simulink model "powerwindow04"  (Simulink 10.0)
settings: Solver=ode23tb  StartTime=0.0  StopTime=inf  FixedStep=1e-4  RelTol=1e-2  EnableMultiTasking=on
libraries: powerlib x11, simulink x6, powerwindowlibphys x1, dspquant2 x1
Description:
  | Simulink(R) Power Window Controller With Data Acquisition Effects
  | 
  | In moving to an implementation, additional effects that may affect the control have to be
  | accounted for. This model includes phenomena such as signal conditioning to measure
  | the armature current and quantization of the measurement.
  | 
  | You must install SimMechanics(TM), SimPowerSystems(TM), DSP System Toolbox(TM), and Simulink(R) Fixed Point(TM) to run this power window demo.
settings Model: Creator=The MathWorks Inc.  LastModifiedBy=bhisma  ExtModeAutoUpdateStatusClock=off
settings DataIOCC: LimitDataPoints=on  SignalLoggingSaveFormat=ModelDataLogs  SignalLoggingName=sigsOut
settings OptimizationCC: BooleanDataType=off  ExpressionDepthLimit=2147483647  InitFltsAndDblsToZero=on
settings DebuggingCC: SaveWithParameterizedLinksMsg=none  CheckExecutionContextPreStartOutputMsg=on  CheckExecutionContextRuntimeOutputMsg=on  SignalResolutionControl=TryResolveAllWithWarning  MultiTaskDSMMsg=warning  MultiTaskCondExecSysMsg=none  ParameterPrecisionLossMsg=none  FcnCallInpInsideContextMsg=warning  StateNameClashWarn=warning
settings SFSimCC: SimParseCustomCode=off
settings GRTTargetCC: TargetFcnLib=ansi_tfl_tmw.mat  GeneratePreprocessorConditionals=Disable all
settings ConfigComp: CovExternalEMLEnable=off
settings SimscapeCC: SimscapeNormalizeSystem=off
settings SimMechanicsCC: WarnOnRedundantConstraints=off  VisOnUpdateDiagram=on

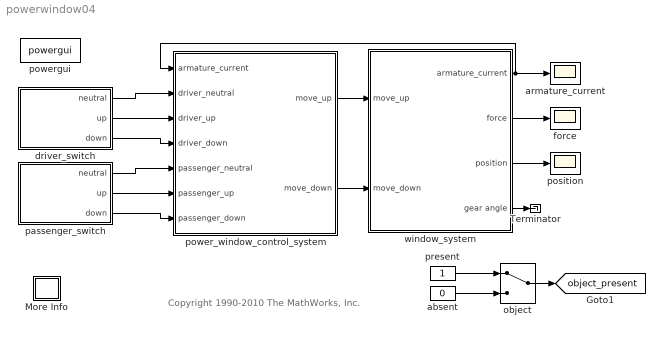
== system powerwindow04 ==
  note: Copyright 1990-2010 The MathWorks, Inc.
  More Info : Subsystem
      settings: OpenFcn=showdemo(bdroot(gcb))
      mask Display: disp('?')
  Terminator : Terminator
  absent : Constant  Value=0
  armature_current : Scope
  driver_switch : Subsystem
  force : Scope
  object : ManualSwitch
  passenger_switch : Subsystem
  position : Scope
  power_window_control_system : Subsystem
  powergui : powerlib/powergui  SimulationMode=Continuous  SampleTime=50e-6  frequency=60  Iterations=50  frequencyindice=0  Pbase=100e6  ErrMax=1e-4  UnitsV=kV  UnitsW=MW  buscounter=0  FunctionMessages=off  echomessages=off  EnableUseOfTLC=off  CurrentSourceSwitches=off  DisableSnubberDevices=off  DisableRonSwitches=off  DisableVfSwitches=off  DisplayEquations=off  AutomaticDiscreteSolvers=off  SolverType=Tustin  Interpol=off  ExternalGateDelay=off  methode=off  Ts=0  x0status=blocks  SPID=off  SwTol=0  HookPort=off  NonlinearTolerance=1e-4  nMaxIteration=100  ContinueOnMaxIteration=off  RestoreLinks=warning  ResistiveCurrentMeasurement=off  Frange=[0:2:500]  Ylog=off  Xlog=on  ShowGrid=off  save=off  variable=ZData  structure=0  ZoomFFT=on  StartTime=0.0  cycles=1  DisplayStyle=1  fundamental=60  FreqAxis=off  MaxFrequency=1000  frequencyindicesteady=1  RmsSteady=1  display=off
      settings: SourceProductName=Simscape Electrical
  present : Constant
  window_system : Subsystem
  tag scope: object_present=global
  wires:
  driver_switch/1(neutral) -> power_window_control_system/2(driver_neutral)
  driver_switch/2(up) -> power_window_control_system/3(driver_up)
  driver_switch/3(down) -> power_window_control_system/4(driver_down)
  passenger_switch/1(neutral) -> power_window_control_system/5(passenger_neutral)
  passenger_switch/2(up) -> power_window_control_system/6(passenger_up)
  passenger_switch/3(down) -> power_window_control_system/7(passenger_down)
  power_window_control_system/1(move_up) -> window_system/1(move_up)
  power_window_control_system/2(move_down) -> window_system/2(move_down)
  window_system/1(armature_current) -> armature_current/1, power_window_control_system/1(armature_current)
  present/1 -> object/1
  absent/1 -> object/2
  object/1 -> [object_present]
  window_system/4(gear angle) -> Terminator/1
  window_system/2(force) -> force/1
  window_system/3(position) -> position/1

== system powerwindow04/More Info ==

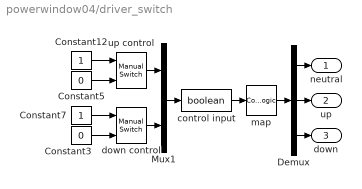
== system powerwindow04/driver_switch ==
  Constant12 : Constant
  Constant3 : Constant  Value=0
  Constant5 : Constant  Value=0
  Constant7 : Constant
  Demux : Demux  Outputs=3
  Mux1 : Mux  Inputs=2
  control input : DataTypeConversion  OutDataTypeStr=boolean  SaturateOnIntegerOverflow=on  RndMeth=Zero
  down control : simulink/Signal Routing/Manual Switch  SystemSampleTime=-1  sw=0  action=0  varsize=off
      settings: SourceProductName=Simulink  SourceProductBaseCode=SL
  map : CombinatorialLogic  TruthTable=[1 0 0;0 0 1;0 1 0;1 0 0]
  up control : simulink/Signal Routing/Manual Switch  SystemSampleTime=-1  sw=1  action=0  varsize=off
      settings: SourceProductName=Simulink  SourceProductBaseCode=SL
  neutral : Outport
  up : Outport  Port=2
  down : Outport  Port=3
  wires:
  control input/1 -> map/1
  Constant12/1 -> up control/1
  Constant5/1 -> up control/2
  Constant7/1 -> down control/1
  Constant3/1 -> down control/2
  down control/1 -> Mux1/2
  Mux1/1 -> control input/1
  up control/1 -> Mux1/1
  map/1 -> Demux/1
  Demux/1 -> neutral/1
  Demux/2 -> up/1
  Demux/3 -> down/1

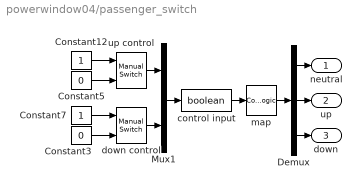
== system powerwindow04/passenger_switch ==
  Constant12 : Constant
  Constant3 : Constant  Value=0
  Constant5 : Constant  Value=0
  Constant7 : Constant
  Demux : Demux  Outputs=3
  Mux1 : Mux  Inputs=2
  control input : DataTypeConversion  OutDataTypeStr=boolean  SaturateOnIntegerOverflow=on  RndMeth=Zero
  down control : simulink/Signal Routing/Manual Switch  SystemSampleTime=-1  sw=0  action=0  varsize=off
      settings: SourceProductName=Simulink  SourceProductBaseCode=SL
  map : CombinatorialLogic  TruthTable=[1 0 0;0 0 1;0 1 0;1 0 0]
  up control : simulink/Signal Routing/Manual Switch  SystemSampleTime=-1  sw=0  action=0  varsize=off
      settings: SourceProductName=Simulink  SourceProductBaseCode=SL
  neutral : Outport
  up : Outport  Port=2
  down : Outport  Port=3
  wires:
  Demux/3 -> down/1
  Demux/2 -> up/1
  Demux/1 -> neutral/1
  map/1 -> Demux/1
  up control/1 -> Mux1/1
  Mux1/1 -> control input/1
  down control/1 -> Mux1/2
  Constant3/1 -> down control/2
  Constant7/1 -> down control/1
  Constant5/1 -> up control/2
  Constant12/1 -> up control/1
  control input/1 -> map/1

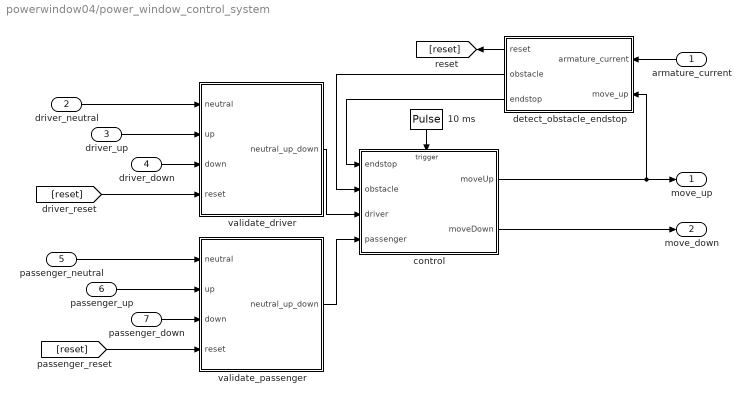
== system powerwindow04/power_window_control_system ==
  armature_current : Inport
  driver_neutral : Inport  Port=2
  driver_up : Inport  Port=3
  driver_down : Inport  Port=4
  passenger_neutral : Inport  Port=5
  passenger_up : Inport  Port=6
  passenger_down : Inport  Port=7
  10 ms : DiscretePulseGenerator  SampleTime=10e-3
  control : Stateflow chart  TreatAsAtomicUnit=on
  detect_obstacle_endstop : Subsystem
  validate_driver : Subsystem
  validate_passenger : Subsystem
  move_up : Outport
  move_down : Outport  Port=2
  wires:
  detect_obstacle_endstop/2(obstacle) -> control/2(obstacle)
  detect_obstacle_endstop/3(endstop) -> control/1(endstop)
  detect_obstacle_endstop/1(reset) -> [reset]
  armature_current/1 -> detect_obstacle_endstop/1(armature_current)
  10 ms/1 -> control/Trigger
  control/1(moveUp) -> move_up/1, detect_obstacle_endstop/2(move_up)
  control/2(moveDown) -> move_down/1
  driver_neutral/1 -> validate_driver/1(neutral)
  driver_up/1 -> validate_driver/2(up)
  driver_down/1 -> validate_driver/3(down)
  [reset] -> validate_driver/4(reset)
  passenger_neutral/1 -> validate_passenger/1(neutral)
  passenger_up/1 -> validate_passenger/2(up)
  passenger_down/1 -> validate_passenger/3(down)
  [reset] -> validate_passenger/4(reset)
  validate_driver/1(neutral_up_down) -> control/3(driver)
  validate_passenger/1(neutral_up_down) -> control/4(passenger)

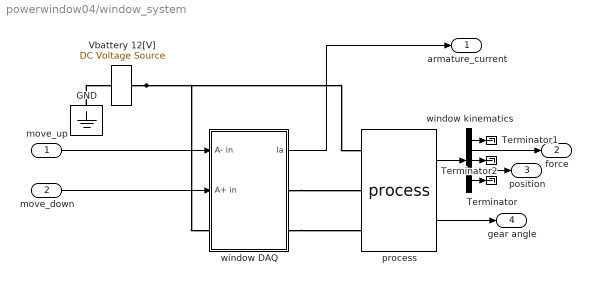
== system powerwindow04/window_system ==
  move_up : Inport
  move_down : Inport  Port=2
  GND : powerlib/Elements/Ground  PhysicalDomain=powersysdomain  SubClassName=unknown  LeftPortType=p1  RightPortType=p1  LConnTagsString=a
      settings: SourceProductName=Simscape Electrical
  Terminator : Terminator
  Terminator1 : Terminator
  Terminator2 : Terminator
  Vbattery 12[V] : powerlib/Electrical Sources/DC Voltage Source  SystemSampleTime=-1  Amplitude=12  Measurements=None
      settings: SourceProductName=Simscape Electrical
  process : powerwindowlibphys/process  SystemSampleTime=-1
  window DAQ : Subsystem
  window kinematics : Demux  Outputs=[1,1,2,1,4]
  armature_current : Outport
  force : Outport  Port=2
  position : Outport  Port=3
  gear angle : Outport  Port=4
  wires:
  window kinematics/2 -> force/1
  window kinematics/1 -> Terminator1/1
  window kinematics/4 -> position/1
  window kinematics/5 -> Terminator/1
  window kinematics/3 -> Terminator2/1
  move_up/1 -> window DAQ/1(A- in)
  move_down/1 -> window DAQ/2(A+ in)
  window DAQ/1(Ia) -> armature_current/1
  process/1 -> window kinematics/1
  process/2 -> gear angle/1
  connections:
  GND/LConn1 -- Vbattery 12[V]/LConn1
  Vbattery 12[V]/RConn1 -- window DAQ/LConn1 -- process/LConn1
  window DAQ/RConn1 -- process/LConn2
  window DAQ/RConn2 -- process/LConn3

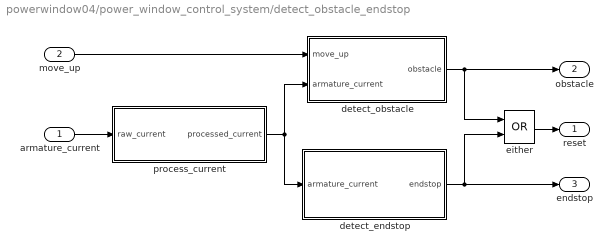
== system powerwindow04/power_window_control_system/detect_obstacle_endstop ==
  armature_current : Inport
  move_up : Inport  Port=2
  detect_endstop : Subsystem
  detect_obstacle : Subsystem
  either : Logic  Operator=OR
  process_current : Subsystem
  reset : Outport
  obstacle : Outport  Port=2
  endstop : Outport  Port=3
  wires:
  armature_current/1 -> process_current/1(raw_current)
  detect_obstacle/1(obstacle) -> either/1, obstacle/1
  detect_endstop/1(endstop) -> endstop/1, either/2
  either/1 -> reset/1
  move_up/1 -> detect_obstacle/1(move_up)
  process_current/1(processed_current) -> detect_endstop/1(armature_current), detect_obstacle/2(armature_current)

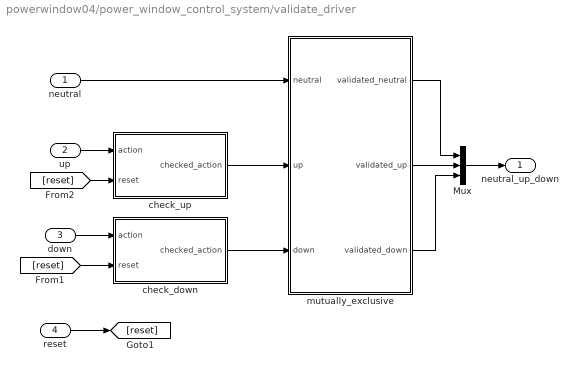
== system powerwindow04/power_window_control_system/validate_driver ==
  neutral : Inport
  up : Inport  Port=2
  down : Inport  Port=3
  reset : Inport  Port=4
  Mux : Mux  Inputs=3
  check_down : Subsystem
  check_up : Subsystem
  mutually_exclusive : Subsystem
  neutral_up_down : Outport
  wires:
  Mux/1 -> neutral_up_down/1
  reset/1 -> [reset]
  [reset] -> check_down/2(reset)
  [reset] -> check_up/2(reset)
  check_up/1(checked_action) -> mutually_exclusive/2(up)
  neutral/1 -> mutually_exclusive/1(neutral)
  up/1 -> check_up/1(action)
  down/1 -> check_down/1(action)
  mutually_exclusive/1(validated_neutral) -> Mux/1
  mutually_exclusive/2(validated_up) -> Mux/2
  mutually_exclusive/3(validated_down) -> Mux/3
  check_down/1(checked_action) -> mutually_exclusive/3(down)

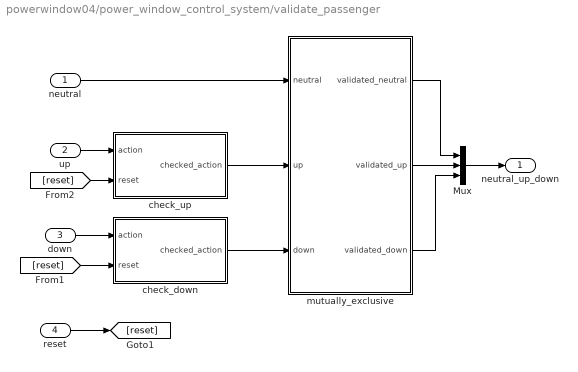
== system powerwindow04/power_window_control_system/validate_passenger ==
  neutral : Inport
  up : Inport  Port=2
  down : Inport  Port=3
  reset : Inport  Port=4
  Mux : Mux  Inputs=3
  check_down : Subsystem
  check_up : Subsystem
  mutually_exclusive : Subsystem
  neutral_up_down : Outport
  wires:
  Mux/1 -> neutral_up_down/1
  reset/1 -> [reset]
  [reset] -> check_down/2(reset)
  [reset] -> check_up/2(reset)
  check_up/1(checked_action) -> mutually_exclusive/2(up)
  neutral/1 -> mutually_exclusive/1(neutral)
  up/1 -> check_up/1(action)
  down/1 -> check_down/1(action)
  mutually_exclusive/1(validated_neutral) -> Mux/1
  mutually_exclusive/2(validated_up) -> Mux/2
  mutually_exclusive/3(validated_down) -> Mux/3
  check_down/1(checked_action) -> mutually_exclusive/3(down)

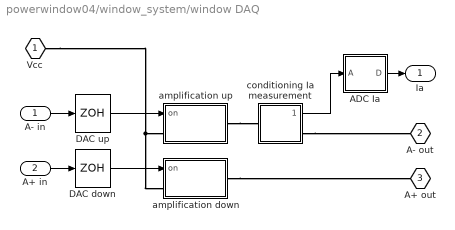
== system powerwindow04/window_system/window DAQ ==
  A- in : Inport
  A+ in : Inport  Port=2
  ADC Ia : Subsystem  mask(AD Converter){Ts=0.01, peak=3.5, Td=0.005, bits=8}
      mask prompts: Ts "sample time (-1 for inherited)"; Td "delay (-1 for inherited)"
      mask help: Analog (A) to digital (D) converter with sample rate, conversion delay, range, and number of bits used for conversion.
      mask Display:
      | plot([0.5 1.5 1.5 2.5 2.5 3.5 3.5 4.5], [0 0 1 1 2 2 3 3])
      | plot([0 3], [0 3])
  DAC down : ZeroOrderHold  SampleTime=0.01
  DAC up : ZeroOrderHold  SampleTime=0.01
  amplification down : Subsystem
  amplification up : Subsystem
  conditioning Ia measurement : Subsystem
  Vcc : PMIOPort  Side=Left
  A- out : PMIOPort  Port=2  Side=Right
  A+ out : PMIOPort  Port=3  Side=Right
  Ia : Outport
  wires:
  DAC up/1 -> amplification up/1(on)
  DAC down/1 -> amplification down/1(on)
  conditioning Ia measurement/1(Vmeas) -> ADC Ia/1(A)
  ADC Ia/1(D) -> Ia/1
  A- in/1 -> DAC up/1
  A+ in/1 -> DAC down/1
  connections:
  amplification up/RConn1 -- conditioning Ia measurement/LConn1
  conditioning Ia measurement/RConn1 -- A- out/RConn1
  amplification down/RConn1 -- A+ out/RConn1
  Vcc/RConn1 -- amplification down/LConn1 -- amplification up/LConn1

== system powerwindow04/power_window_control_system/detect_obstacle_endstop/detect_endstop ==
  armature_current : Inport
  current_limit : simulink/Logic and Bit Operations/Compare To Constant  SystemSampleTime=-1  relop=>  const=15  LogicOutDataTypeMode=uint8  ZeroCross=off
  passenger control : DataTypeConversion  OutDataTypeStr=boolean  SaturateOnIntegerOverflow=on  RndMeth=Zero
  endstop : Outport
  wires:
  passenger control/1 -> endstop/1
  current_limit/1 -> passenger control/1
  armature_current/1 -> current_limit/1

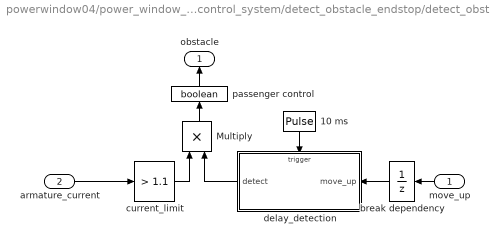
== system powerwindow04/power_window_control_system/detect_obstacle_endstop/detect_obstacle ==
  move_up : Inport
  armature_current : Inport  Port=2
  10 ms : DiscretePulseGenerator  SampleTime=10e-3
  Multiply : Product  Inputs=**  OutDataTypeStr=Inherit: Same as first input
  break dependency : UnitDelay  SampleTime=0.01  HasFrameUpgradeWarning=on
  current_limit : simulink/Logic and Bit Operations/Compare To Constant  SystemSampleTime=-1  relop=>  const=1.1  LogicOutDataTypeMode=uint8  ZeroCross=off
  delay_detection : Stateflow chart  TreatAsAtomicUnit=on
  passenger control : DataTypeConversion  OutDataTypeStr=boolean  SaturateOnIntegerOverflow=on  RndMeth=Zero
  obstacle : Outport
  wires:
  passenger control/1 -> obstacle/1
  break dependency/1 -> delay_detection/1(move_up)
  10 ms/1 -> delay_detection/Trigger
  Multiply/1 -> passenger control/1
  move_up/1 -> break dependency/1
  armature_current/1 -> current_limit/1
  delay_detection/1(" detect") -> Multiply/2
  current_limit/1 -> Multiply/1

== system powerwindow04/power_window_control_system/detect_obstacle_endstop/process_current ==
  raw_current : Inport
  3.5 / (2^(bits-1)) : Gain  Gain=0.02734375  OutDataTypeStr=fixdt(1,16,6)
  Abs : Abs
  gain : Gain  Gain=5  OutDataTypeStr=fixdt(1,16,5)
  processed_current : Outport
  wires:
  raw_current/1 -> 3.5 / (2^(bits-1))/1
  Abs/1 -> processed_current/1
  gain/1 -> Abs/1
  3.5 / (2^(bits-1))/1 -> gain/1

== system powerwindow04/power_window_control_system/validate_driver/check_down ==
  action : Inport
  reset : Inport  Port=2
  allow_action : Logic
  overrule : Logic  Operator=NOT
  checked_action : Outport
  wires:
  reset/1 -> overrule/1
  allow_action/1 -> checked_action/1
  action/1 -> allow_action/1
  overrule/1 -> allow_action/2

== system powerwindow04/power_window_control_system/validate_driver/check_up ==
  action : Inport
  reset : Inport  Port=2
  allow_action : Logic
  overrule : Logic  Operator=NOT
  checked_action : Outport
  wires:
  overrule/1 -> allow_action/2
  action/1 -> allow_action/1
  allow_action/1 -> checked_action/1
  reset/1 -> overrule/1

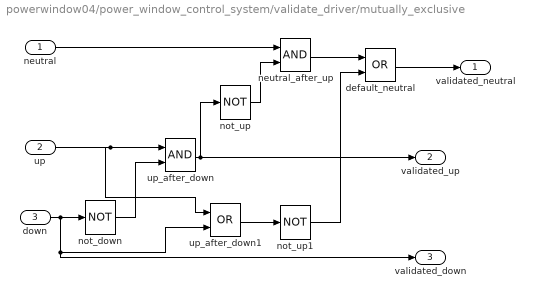
== system powerwindow04/power_window_control_system/validate_driver/mutually_exclusive ==
  neutral : Inport
  up : Inport  Port=2
  down : Inport  Port=3
  default_neutral : Logic  Operator=OR
  neutral_after_up : Logic
  not_down : Logic  Operator=NOT
  not_up : Logic  Operator=NOT
  not_up1 : Logic  Operator=NOT
  up_after_down : Logic
  up_after_down1 : Logic  Operator=OR
  validated_neutral : Outport
  validated_up : Outport  Port=2
  validated_down : Outport  Port=3
  wires:
  not_down/1 -> up_after_down/2
  up_after_down/1 -> not_up/1, validated_up/1
  not_up/1 -> neutral_after_up/2
  down/1 -> not_down/1, up_after_down1/2, validated_down/1
  neutral/1 -> neutral_after_up/1
  up/1 -> up_after_down/1, up_after_down1/1
  up_after_down1/1 -> not_up1/1
  neutral_after_up/1 -> default_neutral/1
  default_neutral/1 -> validated_neutral/1
  not_up1/1 -> default_neutral/2

== system powerwindow04/power_window_control_system/validate_passenger/check_down ==
  action : Inport
  reset : Inport  Port=2
  allow_action : Logic
  overrule : Logic  Operator=NOT
  checked_action : Outport
  wires:
  reset/1 -> overrule/1
  allow_action/1 -> checked_action/1
  action/1 -> allow_action/1
  overrule/1 -> allow_action/2

== system powerwindow04/power_window_control_system/validate_passenger/check_up ==
  action : Inport
  reset : Inport  Port=2
  allow_action : Logic
  overrule : Logic  Operator=NOT
  checked_action : Outport
  wires:
  overrule/1 -> allow_action/2
  action/1 -> allow_action/1
  allow_action/1 -> checked_action/1
  reset/1 -> overrule/1

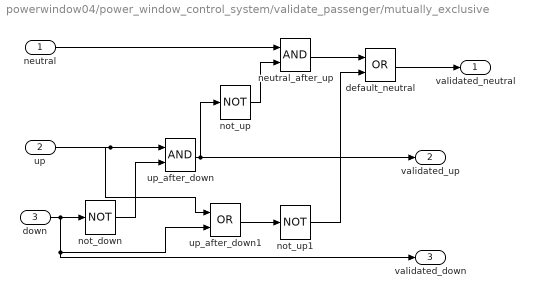
== system powerwindow04/power_window_control_system/validate_passenger/mutually_exclusive ==
  neutral : Inport
  up : Inport  Port=2
  down : Inport  Port=3
  default_neutral : Logic  Operator=OR
  neutral_after_up : Logic
  not_down : Logic  Operator=NOT
  not_up : Logic  Operator=NOT
  not_up1 : Logic  Operator=NOT
  up_after_down : Logic
  up_after_down1 : Logic  Operator=OR
  validated_neutral : Outport
  validated_up : Outport  Port=2
  validated_down : Outport  Port=3
  wires:
  not_down/1 -> up_after_down/2
  up_after_down/1 -> not_up/1, validated_up/1
  not_up/1 -> neutral_after_up/2
  down/1 -> not_down/1, up_after_down1/2, validated_down/1
  neutral/1 -> neutral_after_up/1
  up/1 -> up_after_down/1, up_after_down1/1
  up_after_down1/1 -> not_up1/1
  neutral_after_up/1 -> default_neutral/1
  default_neutral/1 -> validated_neutral/1
  not_up1/1 -> default_neutral/2

== system powerwindow04/window_system/window DAQ/ADC Ia ==
  A : Inport
  Uniform Encoder : dspquant2/Uniform Encoder  peak=peak  bits=bits  otype=Signed integer
      settings: SourceProductName=DSP System Toolbox
  Unit Delay : UnitDelay  SampleTime=Td  HasFrameUpgradeWarning=on
  Zero-Order Hold : ZeroOrderHold  SampleTime=Ts
  D : Outport
  wires:
  Uniform Encoder/1 -> D/1
  A/1 -> Unit Delay/1
  Unit Delay/1 -> Zero-Order Hold/1
  Zero-Order Hold/1 -> Uniform Encoder/1

== system powerwindow04/window_system/window DAQ/amplification down ==
  on : Inport
  Logical Operator : Logic  Operator=NOT
  Terminator1 : Terminator
  Terminator2 : Terminator
  high switch : powerlib/Power Electronics/Ideal Switch  SystemSampleTime=-1  Ron=0.01  Lon=0  IC=0  Rs=1000000  Cs=inf  Measurements=on
      settings: SourceProductName=Simscape Electrical
  low switch : powerlib/Power Electronics/Ideal Switch  SystemSampleTime=-1  Ron=0.01  Lon=0  IC=0  Rs=1000000  Cs=inf  Measurements=on
      settings: SourceProductName=Simscape Electrical
  output Ground1 : powerlib/Elements/Ground  PhysicalDomain=powersysdomain  SubClassName=unknown  LeftPortType=p1  RightPortType=p1  LConnTagsString=a
      settings: SourceProductName=Simscape Electrical
  Vcc : PMIOPort  Side=Left
  pin1 : PMIOPort  Port=2  Side=Right
  wires:
  low switch/1 -> Terminator2/1
  on/1 -> Logical Operator/1, high switch/1
  high switch/1 -> Terminator1/1
  Logical Operator/1 -> low switch/1
  connections:
  high switch/LConn1 -- Vcc/RConn1
  output Ground1/LConn1 -- low switch/LConn1
  low switch/RConn1 -- high switch/RConn1 -- pin1/RConn1

== system powerwindow04/window_system/window DAQ/amplification up ==
  on : Inport
  Logical Operator : Logic  Operator=NOT
  Terminator1 : Terminator
  Terminator2 : Terminator
  high switch : powerlib/Power Electronics/Ideal Switch  SystemSampleTime=-1  Ron=0.01  Lon=0  IC=0  Rs=1000000  Cs=inf  Measurements=on
      settings: SourceProductName=Simscape Electrical
  low switch : powerlib/Power Electronics/Ideal Switch  SystemSampleTime=-1  Ron=0.01  Lon=0  IC=0  Rs=1000000  Cs=inf  Measurements=on
      settings: SourceProductName=Simscape Electrical
  output Ground1 : powerlib/Elements/Ground  PhysicalDomain=powersysdomain  SubClassName=unknown  LeftPortType=p1  RightPortType=p1  LConnTagsString=a
      settings: SourceProductName=Simscape Electrical
  Vcc : PMIOPort  Side=Left
  pin1 : PMIOPort  Port=2  Side=Right
  wires:
  low switch/1 -> Terminator2/1
  on/1 -> high switch/1, Logical Operator/1
  high switch/1 -> Terminator1/1
  Logical Operator/1 -> low switch/1
  connections:
  high switch/RConn1 -- low switch/RConn1 -- pin1/RConn1
  high switch/LConn1 -- Vcc/RConn1
  output Ground1/LConn1 -- low switch/LConn1

== system powerwindow04/window_system/window DAQ/conditioning Ia measurement ==
  R1 : powerlib/Elements/Series RLC Branch  PhysicalDomain=powersysdomain  SubClassName=unknown  LeftPortType=p1  RightPortType=p1  LConnTagsString=__new0  RConnTagsString=__new0  BranchType=R  Resistance=0.18  Inductance=1.0  SetiL0=off  InitialCurrent=0  Capacitance=1.0  Setx0=off  InitialVoltage=0  Measurements=None
      settings: SourceProductName=Simscape Electrical
  measure1 : powerlib/Measurements/Voltage Measurement  SystemSampleTime=-1  PhasorSimulation=off  OutputType=Magnitude  PSBequivalent=0
      settings: SourceProductName=Simscape Electrical
  Vin : PMIOPort  Side=Left
  Vout : PMIOPort  Port=2  Side=Right
  Vmeas : Outport
  wires:
  measure1/1 -> Vmeas/1
  connections:
  measure1/LConn2 -- Vout/RConn1 -- R1/RConn1
  R1/LConn1 -- measure1/LConn1 -- Vin/RConn1

== stateflow chart power_window_control_system/control ==
  settings: executeAtInitialization=1
  state safe
    state driverNeutral
      entry:
      moveUp = 0;
      moveDown = 0;
      state passengerneutral
        entry:
        moveUp = 0;
        moveDown = 0;
      state passengerDown
        entry: moveDown = 1;
        exit: moveDown = 0;
        state iniPassengerDown
        state passengerDown
        state autoPassengerDown
        iniPassengerDown -> (junction 41) : after(100,ticks)
        (junction 41) -> autoPassengerDown [order 1] : [passenger[1]]
        (junction 41) -> safe.driverNeutral.passengerDown.passengerDown [order 2]
      state passengerUp
        entry: moveUp = 1;
        exit: moveUp = 0;
        state iniPassengerUp
        state PassengerUp
        state autoPassengerUp
        iniPassengerUp -> (junction 45) : after(100,ticks)
        (junction 45) -> PassengerUp [order 2]
        (junction 45) -> autoPassengerUp [order 1] : [passenger[1]]
      (default) -> passengerneutral
      passengerneutral -> iniPassengerUp [order 1] : [passenger[2]]
      passengerneutral -> iniPassengerDown [order 2] : [passenger[3]]
      safe.driverNeutral.passengerDown.passengerDown -> passengerneutral : [passenger[1]]
      safe.driverNeutral.passengerDown -> passengerneutral [order 1] : [endstop]
      PassengerUp -> passengerneutral : [passenger[1]]
      passengerUp -> passengerneutral [order 2] : [endstop]
      safe.driverNeutral.passengerDown -> PassengerUp [order 2] : [passenger[2]]
      passengerUp -> safe.driverNeutral.passengerDown.passengerDown [order 1] : [passenger[3]]
    state driverDown
      entry: moveDown = 1;
      exit: moveDown = 0;
      state iniDriverDown
      state autoDriverDown
      state DriverDown
      iniDriverDown -> (junction 49) : after(100,ticks)
      (junction 49) -> autoDriverDown [order 1] : [driver[1]]
      (junction 49) -> DriverDown [order 2]
    state driverUp
      entry: moveUp = 1;
      exit: moveUp = 0;
      state iniDriverUp
      state DriverUp
      state autoDriverUp
      iniDriverUp -> (junction 53) : after(100,ticks)
      (junction 53) -> DriverUp [order 2]
      (junction 53) -> autoDriverUp [order 1] : [driver[1]]
    (default) -> driverNeutral
    driverNeutral -> iniDriverDown [order 2] : [driver[3]]
    DriverDown -> driverNeutral : [driver[1]]
    driverDown -> driverNeutral [order 1] : [endstop]
    DriverUp -> driverNeutral : [driver[1]]
    driverUp -> driverNeutral [order 2] : [endstop]
    driverNeutral -> iniDriverUp [order 1] : [driver[2]]
    driverDown -> DriverUp [order 2] : [driver[2]]
    driverUp -> DriverDown [order 1] : [driver[3]]
  state emergencyDown
    entry:
    moveUp = 0;
    moveDown = 1;
  emergencyDown -> passengerneutral : [endstop | after(100,ticks)]
  (default) -> safe
  safe -> emergencyDown : [obstacle]
  data: moveUp output double; moveDown output double; endstop input boolean; obstacle input boolean; driver input boolean size=3; passenger input boolean size=3
  events: ticks input EITHER_EDGE_EVENT

== stateflow chart power_window_control_system/detect_obstacle_endstop/detect_obstacle/delay_detection ==
  settings: executeAtInitialization=1
  state off
  state hold
  state detect
  (default) -> off
  off -> hold : [move_up]
  detect -> off : [~move_up]
  hold -> off [order 2] : [~move_up]
  hold -> detect [order 1] : [after(100,ticks)]
  data: detect output unknown; move_up input boolean
  events: ticks input EITHER_EDGE_EVENT
